simulink model "practica2simulink"  (R2024b)
settings: Solver=VariableStepAuto  StartTime=0.0  StopTime=3  RelTol=1e-3
values from neighbouring files (symbols this model uses):
  Beq = 4.3    [practica1.m]    (also in tarea1.m)
  Bp = 0.0024    [practica1.m]    (also in tarea1.m)
  Fc = 0    [practica1.m]    (also in tarea1.m)
  g = 9.81    [practica1.m]    (also in tarea1.m)
  Ip = 0.0079    [practica1.m]    (also in tarea1.m)
  lp = 0.3302    [practica1.m]    (also in tarea1.m)
  Mc = 0.7031    [practica1.m]    (also in tarea1.m)
  Mp = 0.23    [practica1.m]    (also in tarea1.m)
settings Model: LastModifiedBy=karla

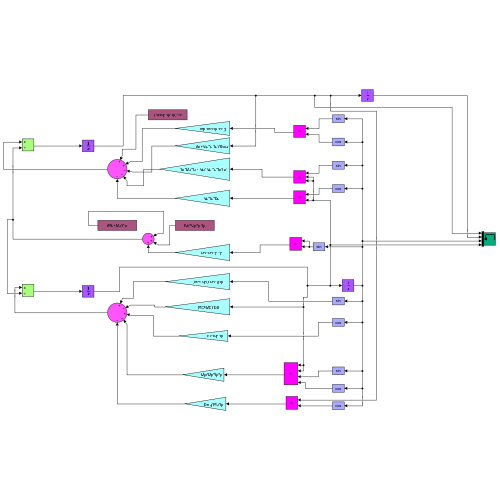
[thumbnail: Simulink's stored preview of the top-level diagram]
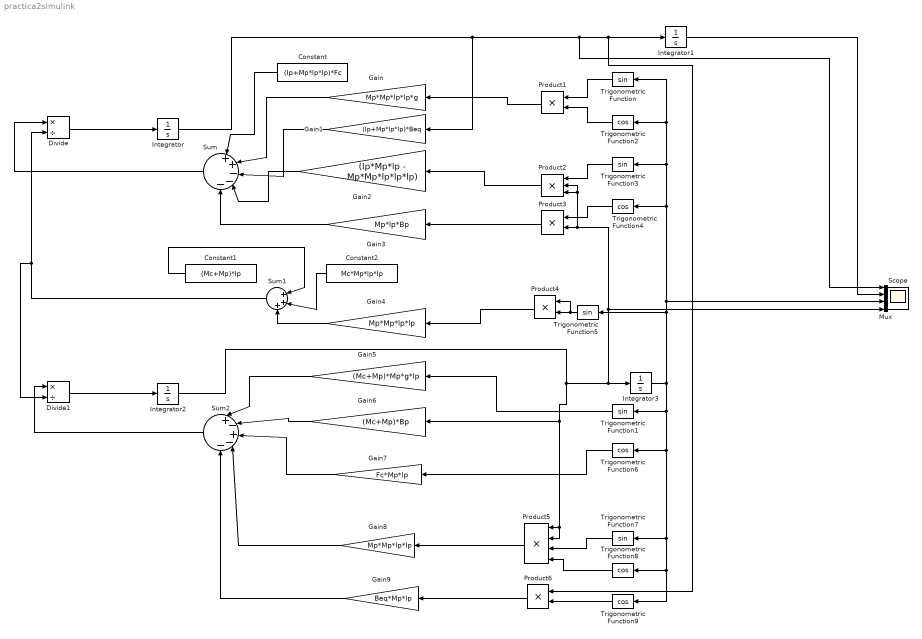
== system practica2simulink ==
  Constant : Constant  Value=(Ip+Mp*lp*lp)*Fc
  Constant1 : Constant  Value=(Mc+Mp)*Ip
  Constant2 : Constant  Value=Mc*Mp*lp*lp
  Divide : Product  Inputs=*/
  Divide1 : Product  Inputs=*/
  Gain : Gain  Gain=Mp*Mp*lp*lp*g
  Gain1 : Gain  Gain=(Ip+Mp*lp*lp)*Beq
  Gain2 : Gain  Gain=(Ip*Mp*lp - Mp*Mp*lp*lp*lp)
  Gain3 : Gain  Gain=Mp*lp*Bp
  Gain4 : Gain  Gain=Mp*Mp*lp*lp
  Gain5 : Gain  Gain=(Mc+Mp)*Mp*g*lp
  Gain6 : Gain  Gain=(Mc+Mp)*Bp
  Gain7 : Gain  Gain=Fc*Mp*lp
  Gain8 : Gain  Gain=Mp*Mp*lp*lp
  Gain9 : Gain  Gain=Beq*Mp*lp
  Integrator : Integrator
  Integrator1 : Integrator
  Integrator2 : Integrator
  Integrator3 : Integrator  InitialCondition=pi/180
  Mux : Mux
  Product{1,3..4,6} (4 alike) : Product
  Product2 : Product  Inputs=3
  Product5 : Product  Inputs=4
  Scope : Scope
  Sum : Sum  Inputs=|+|+|-|-|-
  Sum1 : Sum  Inputs=|+++
  Sum2 : Sum  Inputs=|+|-|+|-|-
  Trigonometric Function{,1,3,5,7} (5 alike) : Trigonometry
  Trigonometric Function{2,4,6,8..9} (5 alike) : Trigonometry  Operator=cos
  wires:
  Gain5/1 -> Sum2/1
  Product2/1 -> Gain2/1
  Sum2/1 -> Divide1/1
  Gain8/1 -> Sum2/4
  Gain7/1 -> Sum2/3
  Trigonometric Function9/1 -> Product6/2
  Constant/1 -> Sum/1
  Product4/1 -> Gain4/1
  Trigonometric Function6/1 -> Gain7/1
  Integrator2/1 -> Product5/1, Product5/2, Gain6/1, Product2/2, Product2/3, Product3/2, Mux/4, Integrator3/1
  Trigonometric Function8/1 -> Product5/4
  Product6/1 -> Gain9/1
  Sum1/1 -> Divide1/2, Divide/2
  Trigonometric Function7/1 -> Product5/3
  Gain4/1 -> Sum1/3
  Integrator3/1 -> Trigonometric Function/1, Trigonometric Function2/1, Trigonometric Function3/1, Trigonometric Function4/1, Mux/3, Trigonometric Function5/1, Trigonometric Function9/1, Trigonometric Function8/1, Trigonometric Function7/1, Trigonometric Function6/1, Trigonometric Function1/1
  Divide1/1 -> Integrator2/1
  Product5/1 -> Gain8/1
  Gain2/1 -> Sum/4
  Integrator/1 -> Mux/1, Product6/1, Integrator1/1, Gain1/1
  Trigonometric Function/1 -> Product1/1
  Gain9/1 -> Sum2/5
  Gain/1 -> Sum/2
  Integrator1/1 -> Mux/2
  Mux/1 -> Scope/1
  Constant2/1 -> Sum1/2
  Divide/1 -> Integrator/1
  Product3/1 -> Gain3/1
  Trigonometric Function3/1 -> Product2/1
  Gain3/1 -> Sum/5
  Constant1/1 -> Sum1/1
  Gain6/1 -> Sum2/2
  Sum/1 -> Divide/1
  Trigonometric Function4/1 -> Product3/1
  Product1/1 -> Gain/1
  Gain1/1 -> Sum/3
  Trigonometric Function2/1 -> Product1/2
  Trigonometric Function1/1 -> Gain5/1
  Trigonometric Function5/1 -> Product4/1, Product4/2
